simulink model "Switching_05"  (R2022b)
settings: Solver=ode4  StartTime=0.0  StopTime=50  FixedStep=1e-3  MaxStep=1e-3  RelTol=1e-3
undefined symbols (not defined in the file or in its folder): OF_b, OF_k1, OF_k2, p1, p2, p3, PR_k1, PR_k2, PR_k3, theta_d, tolerance_posture, v_sat, w_sat, x_d, y_d
libraries: simulink x18, dspsigops x3
settings Model: Creator=david  LastModifiedBy=david

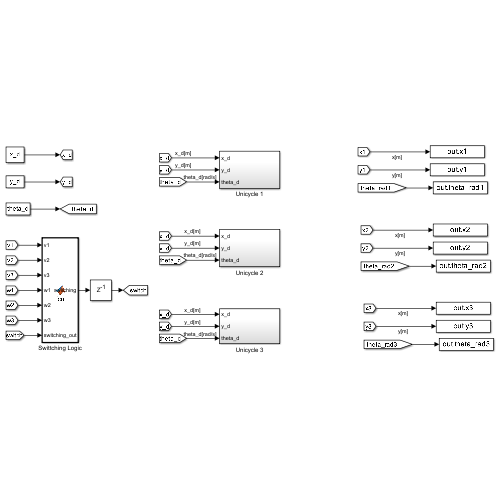
[thumbnail: Simulink's stored preview of the top-level diagram]
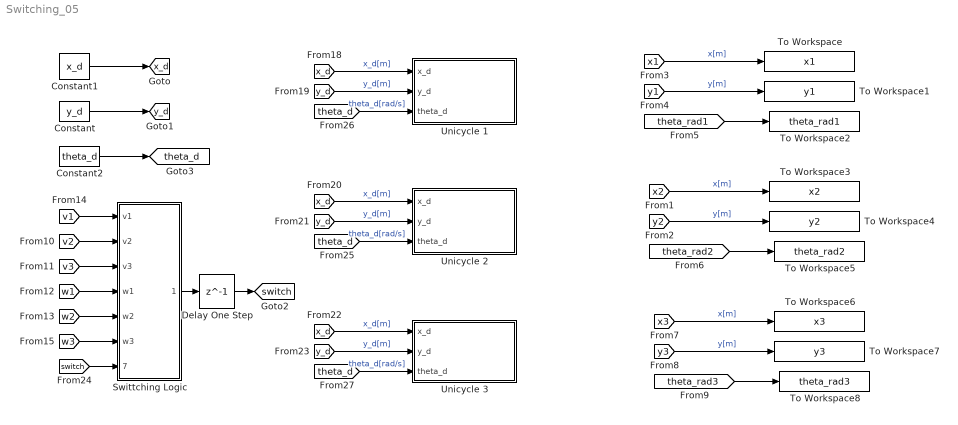
== system Switching_05 ==
  Constant : Constant  Value=y_d
  Constant1 : Constant  Value=x_d
  Constant2 : Constant  Value=theta_d
  Delay One Step : Delay  DelayLength=1
  Swittching Logic : MATLAB Function  TreatAsAtomicUnit=on
  To Workspace : ToWorkspace  VariableName=x1  SaveFormat=Structure With Time  SampleTime=-1
  To Workspace1 : ToWorkspace  VariableName=y1  SaveFormat=Structure With Time  SampleTime=-1
  To Workspace2 : ToWorkspace  VariableName=theta_rad1  SaveFormat=Structure With Time  SampleTime=-1
  To Workspace3 : ToWorkspace  VariableName=x2  SaveFormat=Structure With Time  SampleTime=-1
  To Workspace4 : ToWorkspace  VariableName=y2  SaveFormat=Structure With Time  SampleTime=-1
  To Workspace5 : ToWorkspace  VariableName=theta_rad2  SaveFormat=Structure With Time  SampleTime=-1
  To Workspace6 : ToWorkspace  VariableName=x3  SaveFormat=Structure With Time  SampleTime=-1
  To Workspace7 : ToWorkspace  VariableName=y3  SaveFormat=Structure With Time  SampleTime=-1
  To Workspace8 : ToWorkspace  VariableName=theta_rad3  SaveFormat=Structure With Time  SampleTime=-1
  Unicycle 1 : Subsystem
  Unicycle 2 : Subsystem
  Unicycle 3 : Subsystem
  tag scope: switch=global, theta_d=global, x_d=global, y_d=global
  wires:
  [x1] -> To Workspace/1  "x[m]"
  [y1] -> To Workspace1/1  "y[m]"
  [theta_rad1] -> To Workspace2/1
  [x2] -> To Workspace3/1  "x[m]"
  [y2] -> To Workspace4/1  "y[m]"
  [theta_rad2] -> To Workspace5/1
  [theta_rad3] -> To Workspace8/1
  [y3] -> To Workspace7/1  "y[m]"
  [x3] -> To Workspace6/1  "x[m]"
  Constant1/1 -> [x_d]
  Constant/1 -> [y_d]
  [x_d] -> Unicycle 1/1(x_d)  "x_d[m]"
  [y_d] -> Unicycle 1/2(y_d)  "y_d[m]"
  [y_d] -> Unicycle 2/2(y_d)  "y_d[m]"
  [x_d] -> Unicycle 2/1(x_d)  "x_d[m]"
  [y_d] -> Unicycle 3/2(y_d)  "y_d[m]"
  [x_d] -> Unicycle 3/1(x_d)  "x_d[m]"
  Swittching Logic/1(switching) -> Delay One Step/1
  [switch] -> Swittching Logic/7(switching_out)
  Delay One Step/1 -> [switch]
  Constant2/1 -> [theta_d]
  [theta_d] -> Unicycle 2/3(theta_d)  "theta_d[rad/s]"
  [theta_d] -> Unicycle 1/3(theta_d)  "theta_d[rad/s]"
  [theta_d] -> Unicycle 3/3(theta_d)  "theta_d[rad/s]"
  [w3] -> Swittching Logic/6(w3)
  [v3] -> Swittching Logic/3(v3)
  [w1] -> Swittching Logic/4(w1)
  [w2] -> Swittching Logic/5(w2)
  [v2] -> Swittching Logic/2(v2)
  [v1] -> Swittching Logic/1(v1)

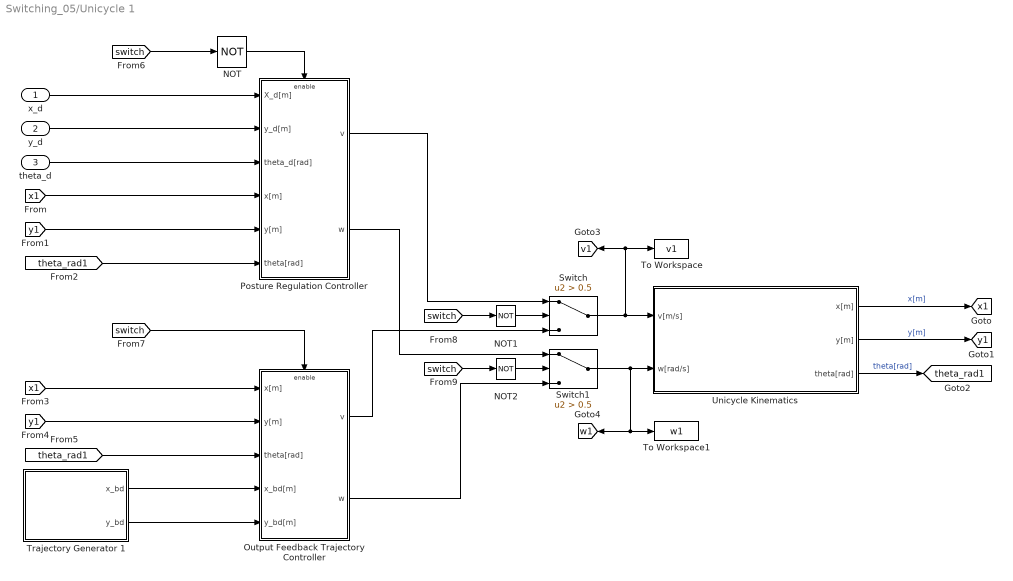
== system Switching_05/Unicycle 1 ==
  x_d : Inport
  y_d : Inport  Port=2
  theta_d : Inport  Port=3
  NOT : Logic  Operator=NOT  IconShape=distinctive  AllPortsSameDT=off  OutDataTypeStr=boolean
  NOT1 : Logic  Operator=NOT  IconShape=distinctive  AllPortsSameDT=off  OutDataTypeStr=boolean
  NOT2 : Logic  Operator=NOT  IconShape=distinctive  AllPortsSameDT=off  OutDataTypeStr=boolean
  Output Feedback Trajectory Controller : Subsystem
  Posture Regulation Controller : Subsystem
  Switch : Switch  Criteria=u2 > Threshold  Threshold=0.5  SaturateOnIntegerOverflow=off  InputSameDT=off
  Switch1 : Switch  Criteria=u2 > Threshold  Threshold=0.5  SaturateOnIntegerOverflow=off  InputSameDT=off
  To Workspace : ToWorkspace  VariableName=v1  SaveFormat=Structure With Time  SampleTime=-1
  To Workspace1 : ToWorkspace  VariableName=w1  SaveFormat=Structure With Time  SampleTime=-1
  Trajectory Generator 1 : Subsystem
  Unicycle Kinematics : Subsystem
  tag scope: theta_rad1=global, v1=global, w1=global, x1=global, y1=global
  wires:
  Unicycle Kinematics/3(theta[rad]) -> [theta_rad1]  "theta[rad]"
  [y1] -> Posture Regulation Controller/5(y[m])
  [theta_rad1] -> Posture Regulation Controller/6(theta[rad])
  Unicycle Kinematics/2(y[m]) -> [y1]  "y[m]"
  [x1] -> Posture Regulation Controller/4(x[m])
  Unicycle Kinematics/1(x[m]) -> [x1]  "x[m]"
  x_d/1 -> Posture Regulation Controller/1(X_d[m])
  y_d/1 -> Posture Regulation Controller/2(y_d[m])
  [theta_rad1] -> Output Feedback Trajectory Controller/3(theta[rad])
  [x1] -> Output Feedback Trajectory Controller/1(x[m])
  [y1] -> Output Feedback Trajectory Controller/2(y[m])
  NOT/1 -> Posture Regulation Controller/Enable
  [switch] -> NOT/1
  [switch] -> Output Feedback Trajectory Controller/Enable
  Posture Regulation Controller/2(w) -> Switch1/1
  Posture Regulation Controller/1(v) -> Switch/1
  Output Feedback Trajectory Controller/2(w) -> Switch1/3
  [switch] -> NOT2/1
  Output Feedback Trajectory Controller/1(v) -> Switch/3
  [switch] -> NOT1/1
  NOT1/1 -> Switch/2
  NOT2/1 -> Switch1/2
  Switch1/1 -> Unicycle Kinematics/2(w[rad/s]), To Workspace1/1, [w1]
  Switch/1 -> Unicycle Kinematics/1(v[m/s]), To Workspace/1, [v1]
  theta_d/1 -> Posture Regulation Controller/3(theta_d[rad])
  Trajectory Generator 1/1(x_bd) -> Output Feedback Trajectory Controller/4(x_bd[m])
  Trajectory Generator 1/2(y_bd) -> Output Feedback Trajectory Controller/5(y_bd[m])

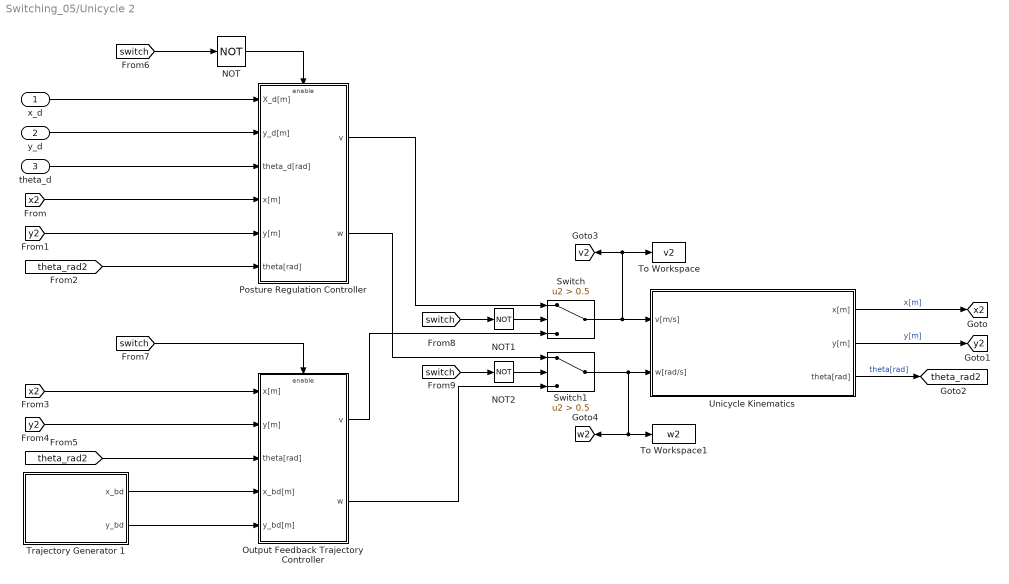
== system Switching_05/Unicycle 2 ==
  x_d : Inport
  y_d : Inport  Port=2
  theta_d : Inport  Port=3
  NOT : Logic  Operator=NOT  IconShape=distinctive  AllPortsSameDT=off  OutDataTypeStr=boolean
  NOT1 : Logic  Operator=NOT  IconShape=distinctive  AllPortsSameDT=off  OutDataTypeStr=boolean
  NOT2 : Logic  Operator=NOT  IconShape=distinctive  AllPortsSameDT=off  OutDataTypeStr=boolean
  Output Feedback Trajectory Controller : Subsystem
  Posture Regulation Controller : Subsystem
  Switch : Switch  Criteria=u2 > Threshold  Threshold=0.5  SaturateOnIntegerOverflow=off  InputSameDT=off
  Switch1 : Switch  Criteria=u2 > Threshold  Threshold=0.5  SaturateOnIntegerOverflow=off  InputSameDT=off
  To Workspace : ToWorkspace  VariableName=v2  SaveFormat=Structure With Time  SampleTime=-1
  To Workspace1 : ToWorkspace  VariableName=w2  SaveFormat=Structure With Time  SampleTime=-1
  Trajectory Generator 1 : Subsystem
  Unicycle Kinematics : Subsystem
  tag scope: theta_rad2=global, v2=global, w2=global, x2=global, y2=global
  wires:
  Unicycle Kinematics/3(theta[rad]) -> [theta_rad2]  "theta[rad]"
  [y2] -> Posture Regulation Controller/5(y[m])
  [theta_rad2] -> Posture Regulation Controller/6(theta[rad])
  Unicycle Kinematics/2(y[m]) -> [y2]  "y[m]"
  [x2] -> Posture Regulation Controller/4(x[m])
  Unicycle Kinematics/1(x[m]) -> [x2]  "x[m]"
  x_d/1 -> Posture Regulation Controller/1(X_d[m])
  y_d/1 -> Posture Regulation Controller/2(y_d[m])
  [theta_rad2] -> Output Feedback Trajectory Controller/3(theta[rad])
  [x2] -> Output Feedback Trajectory Controller/1(x[m])
  [y2] -> Output Feedback Trajectory Controller/2(y[m])
  NOT/1 -> Posture Regulation Controller/Enable
  [switch] -> NOT/1
  [switch] -> Output Feedback Trajectory Controller/Enable
  Posture Regulation Controller/2(w) -> Switch1/1
  Posture Regulation Controller/1(v) -> Switch/1
  Output Feedback Trajectory Controller/2(w) -> Switch1/3
  [switch] -> NOT2/1
  [switch] -> NOT1/1
  NOT1/1 -> Switch/2
  NOT2/1 -> Switch1/2
  Output Feedback Trajectory Controller/1(v) -> Switch/3
  Switch/1 -> Unicycle Kinematics/1(v[m/s]), To Workspace/1, [v2]
  theta_d/1 -> Posture Regulation Controller/3(theta_d[rad])
  Switch1/1 -> Unicycle Kinematics/2(w[rad/s]), [w2], To Workspace1/1
  Trajectory Generator 1/2(y_bd) -> Output Feedback Trajectory Controller/5(y_bd[m])
  Trajectory Generator 1/1(x_bd) -> Output Feedback Trajectory Controller/4(x_bd[m])

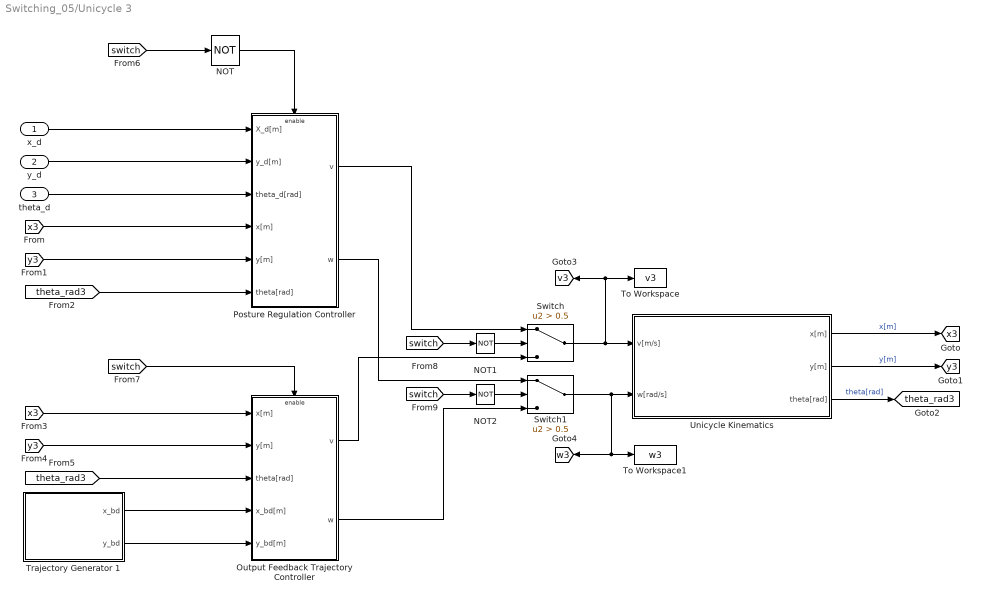
== system Switching_05/Unicycle 3 ==
  x_d : Inport
  y_d : Inport  Port=2
  theta_d : Inport  Port=3
  NOT : Logic  Operator=NOT  IconShape=distinctive  AllPortsSameDT=off  OutDataTypeStr=boolean
  NOT1 : Logic  Operator=NOT  IconShape=distinctive  AllPortsSameDT=off  OutDataTypeStr=boolean
  NOT2 : Logic  Operator=NOT  IconShape=distinctive  AllPortsSameDT=off  OutDataTypeStr=boolean
  Output Feedback Trajectory Controller : Subsystem
  Posture Regulation Controller : Subsystem
  Switch : Switch  Criteria=u2 > Threshold  Threshold=0.5  SaturateOnIntegerOverflow=off  InputSameDT=off
  Switch1 : Switch  Criteria=u2 > Threshold  Threshold=0.5  SaturateOnIntegerOverflow=off  InputSameDT=off
  To Workspace : ToWorkspace  VariableName=v3  SaveFormat=Structure With Time  SampleTime=-1
  To Workspace1 : ToWorkspace  VariableName=w3  SaveFormat=Structure With Time  SampleTime=-1
  Trajectory Generator 1 : Subsystem
  Unicycle Kinematics : Subsystem
  tag scope: theta_rad3=global, v3=global, w3=global, x3=global, y3=global
  wires:
  Unicycle Kinematics/3(theta[rad]) -> [theta_rad3]  "theta[rad]"
  [y3] -> Posture Regulation Controller/5(y[m])
  [theta_rad3] -> Posture Regulation Controller/6(theta[rad])
  Unicycle Kinematics/2(y[m]) -> [y3]  "y[m]"
  [x3] -> Posture Regulation Controller/4(x[m])
  Unicycle Kinematics/1(x[m]) -> [x3]  "x[m]"
  x_d/1 -> Posture Regulation Controller/1(X_d[m])
  y_d/1 -> Posture Regulation Controller/2(y_d[m])
  [theta_rad3] -> Output Feedback Trajectory Controller/3(theta[rad])
  [x3] -> Output Feedback Trajectory Controller/1(x[m])
  [y3] -> Output Feedback Trajectory Controller/2(y[m])
  NOT/1 -> Posture Regulation Controller/Enable
  [switch] -> NOT/1
  [switch] -> Output Feedback Trajectory Controller/Enable
  Posture Regulation Controller/1(v) -> Switch/1
  [switch] -> NOT1/1
  Output Feedback Trajectory Controller/1(v) -> Switch/3
  [switch] -> NOT2/1
  Posture Regulation Controller/2(w) -> Switch1/1
  Output Feedback Trajectory Controller/2(w) -> Switch1/3
  NOT1/1 -> Switch/2
  NOT2/1 -> Switch1/2
  Switch1/1 -> Unicycle Kinematics/2(w[rad/s]), To Workspace1/1, [w3]
  Switch/1 -> Unicycle Kinematics/1(v[m/s]), To Workspace/1, [v3]
  theta_d/1 -> Posture Regulation Controller/3(theta_d[rad])
  Trajectory Generator 1/1(x_bd) -> Output Feedback Trajectory Controller/4(x_bd[m])
  Trajectory Generator 1/2(y_bd) -> Output Feedback Trajectory Controller/5(y_bd[m])

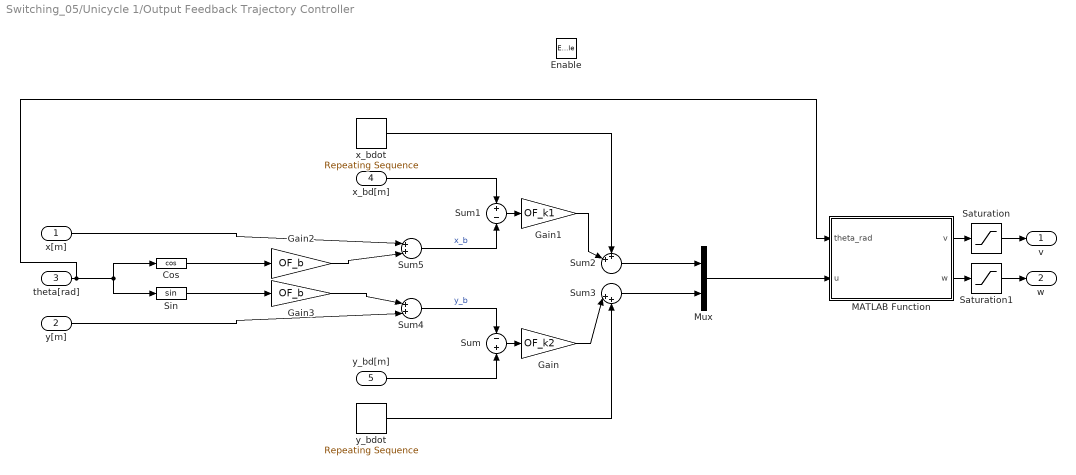
== system Switching_05/Unicycle 1/Output Feedback Trajectory Controller ==
  x[m] : Inport
  y[m] : Inport  Port=2
  theta[rad] : Inport  Port=3
  x_bd[m] : Inport  Port=4
  y_bd[m] : Inport  Port=5
  Enable : EnablePort
  Cos : Trigonometry  Operator=cos
  Gain : Gain  Gain=OF_k2
  Gain1 : Gain  Gain=OF_k1
  Gain2 : Gain  Gain=OF_b
  Gain3 : Gain  Gain=OF_b
  MATLAB Function : MATLAB Function  TreatAsAtomicUnit=on
  Mux : Mux  Inputs=2
  Saturation : Saturate  UpperLimit=v_sat  LowerLimit=-v_sat
  Saturation1 : Saturate  UpperLimit=w_sat  LowerLimit=-w_sat
  Sin : Trigonometry
  Sum : Sum  Inputs=-+
  Sum1 : Sum  Inputs=+-
  Sum2 : Sum  Inputs=++||
  Sum3 : Sum  Inputs=||++
  Sum4 : Sum  Inputs=|++|
  Sum5 : Sum  Inputs=|++|
  x_bdot : simulink/Sources/Repeating Sequence  rep_seq_t=time  rep_seq_y=x_bdot1
  y_bdot : simulink/Sources/Repeating Sequence  rep_seq_t=time  rep_seq_y=y_bdot1
  v : Outport
  w : Outport  Port=2
  wires:
  MATLAB Function/1(v) -> Saturation/1
  MATLAB Function/2(w) -> Saturation1/1
  x_bd[m]/1 -> Sum1/1
  y_bd[m]/1 -> Sum/2
  Mux/1 -> MATLAB Function/2(u)
  Sum2/1 -> Mux/1
  Sum3/1 -> Mux/2
  Sum/1 -> Gain/1
  Sum1/1 -> Gain1/1
  y_bdot/1 -> Sum3/2
  Gain/1 -> Sum3/1
  Gain1/1 -> Sum2/2
  x_bdot/1 -> Sum2/1
  Sum4/1 -> Sum/1  "y_b"
  Sum5/1 -> Sum1/2  "x_b"
  x[m]/1 -> Sum5/1
  y[m]/1 -> Sum4/2
  Cos/1 -> Gain2/1
  Gain3/1 -> Sum4/1
  Gain2/1 -> Sum5/2
  theta[rad]/1 -> Sin/1, Cos/1, MATLAB Function/1(theta_rad)
  Sin/1 -> Gain3/1
  Saturation/1 -> v/1
  Saturation1/1 -> w/1

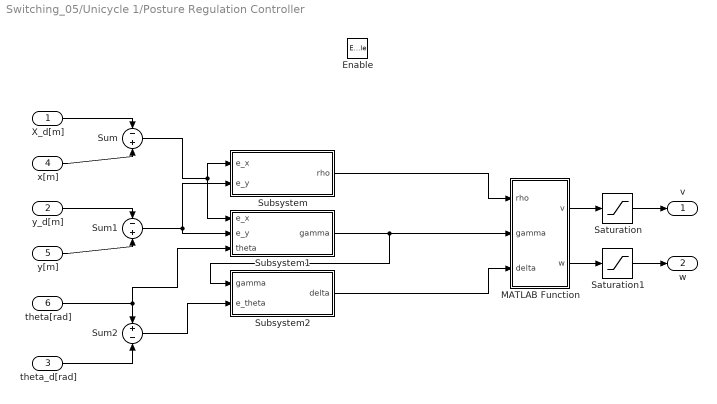
== system Switching_05/Unicycle 1/Posture Regulation Controller ==
  X_d[m] : Inport
  y_d[m] : Inport  Port=2
  theta_d[rad] : Inport  Port=3
  x[m] : Inport  Port=4
  y[m] : Inport  Port=5
  theta[rad] : Inport  Port=6
  Enable : EnablePort
  MATLAB Function : MATLAB Function  TreatAsAtomicUnit=on
  Saturation : Saturate  UpperLimit=v_sat  LowerLimit=-v_sat
  Saturation1 : Saturate  UpperLimit=w_sat  LowerLimit=-w_sat
  Subsystem : Subsystem
  Subsystem1 : Subsystem
  Subsystem2 : Subsystem
  Sum : Sum  Inputs=-+
  Sum1 : Sum  Inputs=-+
  Sum2 : Sum  Inputs=+-
  v : Outport
  w : Outport  Port=2
  wires:
  X_d[m]/1 -> Sum/1
  x[m]/1 -> Sum/2
  y_d[m]/1 -> Sum1/1
  y[m]/1 -> Sum1/2
  Sum1/1 -> Subsystem1/2(e_y), Subsystem/2(e_y)
  Sum2/1 -> Subsystem2/2(e_theta)
  Subsystem1/1(gamma) -> MATLAB Function/2(gamma), Subsystem2/1(gamma)
  Subsystem2/1(delta) -> MATLAB Function/3(delta)
  Subsystem/1(rho) -> MATLAB Function/1(rho)
  Sum/1 -> Subsystem1/1(e_x), Subsystem/1(e_x)
  MATLAB Function/1(v) -> Saturation/1
  MATLAB Function/2(w) -> Saturation1/1
  theta[rad]/1 -> Sum2/1, Subsystem1/3(theta)
  theta_d[rad]/1 -> Sum2/2
  Saturation/1 -> v/1
  Saturation1/1 -> w/1

== system Switching_05/Unicycle 1/Trajectory Generator 1 ==
  To Workspace : ToWorkspace  VariableName=x_bd1  SaveFormat=Structure With Time  SampleTime=-1
  To Workspace1 : ToWorkspace  VariableName=y_bd1  SaveFormat=Structure With Time  SampleTime=-1
  To Workspace2 : ToWorkspace  VariableName=y_d1  SaveFormat=Structure With Time  SampleTime=-1
  To Workspace3 : ToWorkspace  VariableName=x_d1  SaveFormat=Structure With Time  SampleTime=-1
  x_bd1 : simulink/Sources/Repeating Sequence  rep_seq_t=time  rep_seq_y=x_bd1
  x_d1 : simulink/Sources/Repeating Sequence  rep_seq_t=time  rep_seq_y=x_d1
  y_bd1 : simulink/Sources/Repeating Sequence  rep_seq_t=time  rep_seq_y=y_bd1
  y_d1 : simulink/Sources/Repeating Sequence  rep_seq_t=time  rep_seq_y=y_d1
  x_bd : Outport
  y_bd : Outport  Port=2
  wires:
  x_bd1/1 -> x_bd/1, To Workspace/1
  x_d1/1 -> To Workspace3/1
  y_bd1/1 -> y_bd/1, To Workspace1/1
  y_d1/1 -> To Workspace2/1

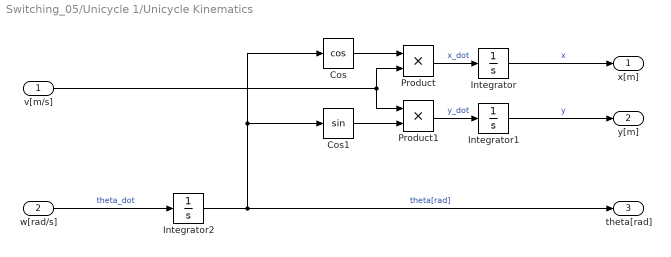
== system Switching_05/Unicycle 1/Unicycle Kinematics ==
  v[m/s] : Inport
  w[rad/s] : Inport  Port=2
  Cos : Trigonometry  Operator=cos
  Cos1 : Trigonometry
  Integrator : Integrator  InitialCondition=p1(1)
  Integrator1 : Integrator  InitialCondition=p1(2)
  Integrator2 : Integrator  InitialCondition=p1(3)
  Product : Product
  Product1 : Product
  x[m] : Outport
  y[m] : Outport  Port=2
  theta[rad] : Outport  Port=3
  wires:
  Integrator/1 -> x[m]/1  "x"
  Integrator1/1 -> y[m]/1  "y"
  w[rad/s]/1 -> Integrator2/1  "theta_dot"
  Integrator2/1 -> Cos/1, Cos1/1, theta[rad]/1  "theta[rad]"
  Product/1 -> Integrator/1  "x_dot"
  Cos1/1 -> Product1/2
  Cos/1 -> Product/1
  v[m/s]/1 -> Product1/1, Product/2
  Product1/1 -> Integrator1/1  "y_dot"

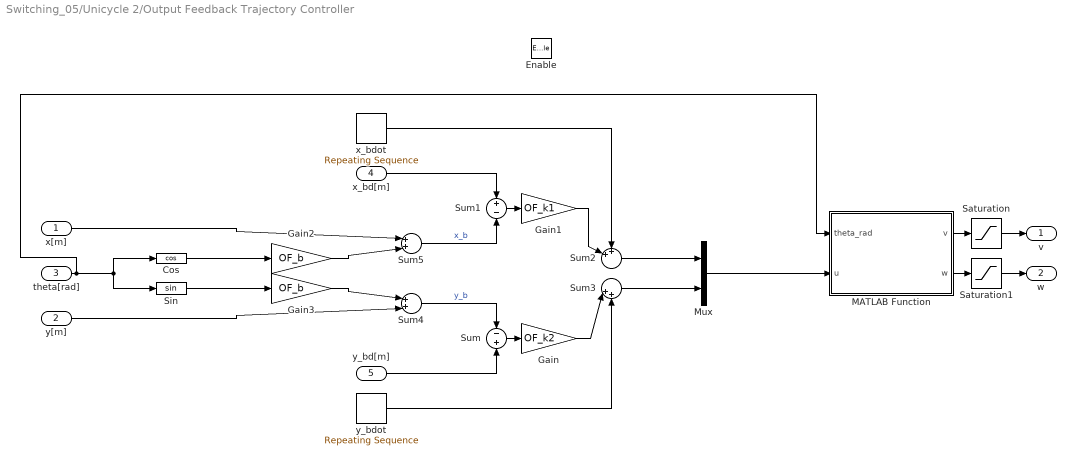
== system Switching_05/Unicycle 2/Output Feedback Trajectory Controller ==
  x[m] : Inport
  y[m] : Inport  Port=2
  theta[rad] : Inport  Port=3
  x_bd[m] : Inport  Port=4
  y_bd[m] : Inport  Port=5
  Enable : EnablePort
  Cos : Trigonometry  Operator=cos
  Gain : Gain  Gain=OF_k2
  Gain1 : Gain  Gain=OF_k1
  Gain2 : Gain  Gain=OF_b
  Gain3 : Gain  Gain=OF_b
  MATLAB Function : MATLAB Function  TreatAsAtomicUnit=on
  Mux : Mux  Inputs=2
  Saturation : Saturate  UpperLimit=v_sat  LowerLimit=-v_sat
  Saturation1 : Saturate  UpperLimit=w_sat  LowerLimit=-w_sat
  Sin : Trigonometry
  Sum : Sum  Inputs=-+
  Sum1 : Sum  Inputs=+-
  Sum2 : Sum  Inputs=++||
  Sum3 : Sum  Inputs=||++
  Sum4 : Sum  Inputs=|++|
  Sum5 : Sum  Inputs=|++|
  x_bdot : simulink/Sources/Repeating Sequence  rep_seq_t=time  rep_seq_y=x_bdot2
  y_bdot : simulink/Sources/Repeating Sequence  rep_seq_t=time  rep_seq_y=y_bdot2
  v : Outport
  w : Outport  Port=2
  wires:
  MATLAB Function/1(v) -> Saturation/1
  MATLAB Function/2(w) -> Saturation1/1
  x_bd[m]/1 -> Sum1/1
  y_bd[m]/1 -> Sum/2
  Mux/1 -> MATLAB Function/2(u)
  Sum2/1 -> Mux/1
  Sum3/1 -> Mux/2
  Sum/1 -> Gain/1
  Sum1/1 -> Gain1/1
  y_bdot/1 -> Sum3/2
  Gain/1 -> Sum3/1
  Gain1/1 -> Sum2/2
  x_bdot/1 -> Sum2/1
  Sum4/1 -> Sum/1  "y_b"
  Sum5/1 -> Sum1/2  "x_b"
  x[m]/1 -> Sum5/1
  y[m]/1 -> Sum4/2
  Cos/1 -> Gain2/1
  Gain3/1 -> Sum4/1
  Gain2/1 -> Sum5/2
  theta[rad]/1 -> Sin/1, Cos/1, MATLAB Function/1(theta_rad)
  Sin/1 -> Gain3/1
  Saturation1/1 -> w/1
  Saturation/1 -> v/1

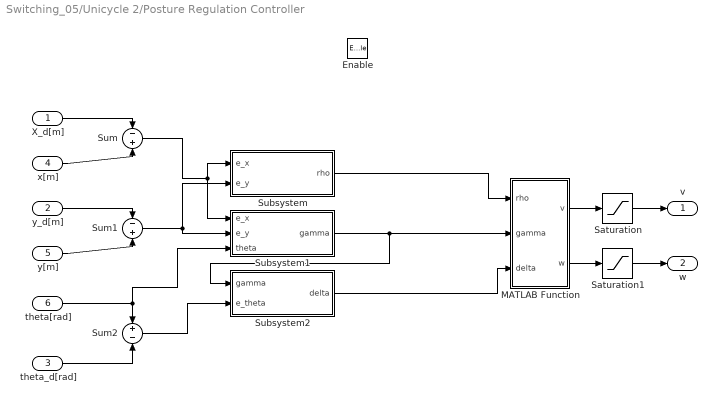
== system Switching_05/Unicycle 2/Posture Regulation Controller ==
  X_d[m] : Inport
  y_d[m] : Inport  Port=2
  theta_d[rad] : Inport  Port=3
  x[m] : Inport  Port=4
  y[m] : Inport  Port=5
  theta[rad] : Inport  Port=6
  Enable : EnablePort
  MATLAB Function : MATLAB Function  TreatAsAtomicUnit=on
  Saturation : Saturate  UpperLimit=v_sat  LowerLimit=-v_sat
  Saturation1 : Saturate  UpperLimit=w_sat  LowerLimit=-w_sat
  Subsystem : Subsystem
  Subsystem1 : Subsystem
  Subsystem2 : Subsystem
  Sum : Sum  Inputs=-+
  Sum1 : Sum  Inputs=-+
  Sum2 : Sum  Inputs=+-
  v : Outport
  w : Outport  Port=2
  wires:
  X_d[m]/1 -> Sum/1
  x[m]/1 -> Sum/2
  y_d[m]/1 -> Sum1/1
  y[m]/1 -> Sum1/2
  Sum1/1 -> Subsystem1/2(e_y), Subsystem/2(e_y)
  Sum2/1 -> Subsystem2/2(e_theta)
  Subsystem1/1(gamma) -> MATLAB Function/2(gamma), Subsystem2/1(gamma)
  Subsystem2/1(delta) -> MATLAB Function/3(delta)
  Subsystem/1(rho) -> MATLAB Function/1(rho)
  Sum/1 -> Subsystem1/1(e_x), Subsystem/1(e_x)
  MATLAB Function/1(v) -> Saturation/1
  MATLAB Function/2(w) -> Saturation1/1
  theta[rad]/1 -> Sum2/1, Subsystem1/3(theta)
  theta_d[rad]/1 -> Sum2/2
  Saturation/1 -> v/1
  Saturation1/1 -> w/1

== system Switching_05/Unicycle 2/Trajectory Generator 1 ==
  To Workspace : ToWorkspace  VariableName=x_bd2  SaveFormat=Structure With Time  SampleTime=-1
  To Workspace1 : ToWorkspace  VariableName=y_bd2  SaveFormat=Structure With Time  SampleTime=-1
  To Workspace2 : ToWorkspace  VariableName=y_d2  SaveFormat=Structure With Time  SampleTime=-1
  To Workspace3 : ToWorkspace  VariableName=x_d2  SaveFormat=Structure With Time  SampleTime=-1
  x_bd2 : simulink/Sources/Repeating Sequence  rep_seq_t=time  rep_seq_y=x_bd2
  x_d2 : simulink/Sources/Repeating Sequence  rep_seq_t=time  rep_seq_y=x_d2
  y_bd2 : simulink/Sources/Repeating Sequence  rep_seq_t=time  rep_seq_y=y_bd2
  y_d2 : simulink/Sources/Repeating Sequence  rep_seq_t=time  rep_seq_y=y_d2
  x_bd : Outport
  y_bd : Outport  Port=2
  wires:
  x_bd2/1 -> x_bd/1, To Workspace/1
  x_d2/1 -> To Workspace3/1
  y_bd2/1 -> y_bd/1, To Workspace1/1
  y_d2/1 -> To Workspace2/1

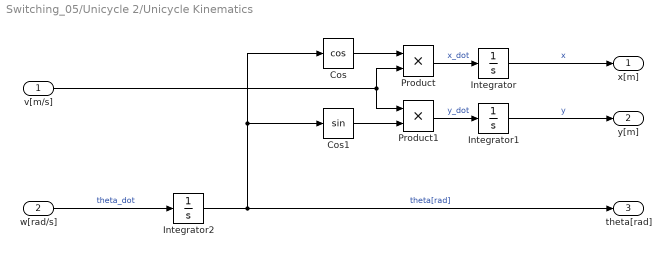
== system Switching_05/Unicycle 2/Unicycle Kinematics ==
  v[m/s] : Inport
  w[rad/s] : Inport  Port=2
  Cos : Trigonometry  Operator=cos
  Cos1 : Trigonometry
  Integrator : Integrator  InitialCondition=p2(1)
  Integrator1 : Integrator  InitialCondition=p2(2)
  Integrator2 : Integrator  InitialCondition=p2(3)
  Product : Product
  Product1 : Product
  x[m] : Outport
  y[m] : Outport  Port=2
  theta[rad] : Outport  Port=3
  wires:
  Integrator/1 -> x[m]/1  "x"
  Integrator1/1 -> y[m]/1  "y"
  w[rad/s]/1 -> Integrator2/1  "theta_dot"
  Integrator2/1 -> Cos/1, Cos1/1, theta[rad]/1  "theta[rad]"
  Product/1 -> Integrator/1  "x_dot"
  Cos1/1 -> Product1/2
  Cos/1 -> Product/1
  v[m/s]/1 -> Product1/1, Product/2
  Product1/1 -> Integrator1/1  "y_dot"

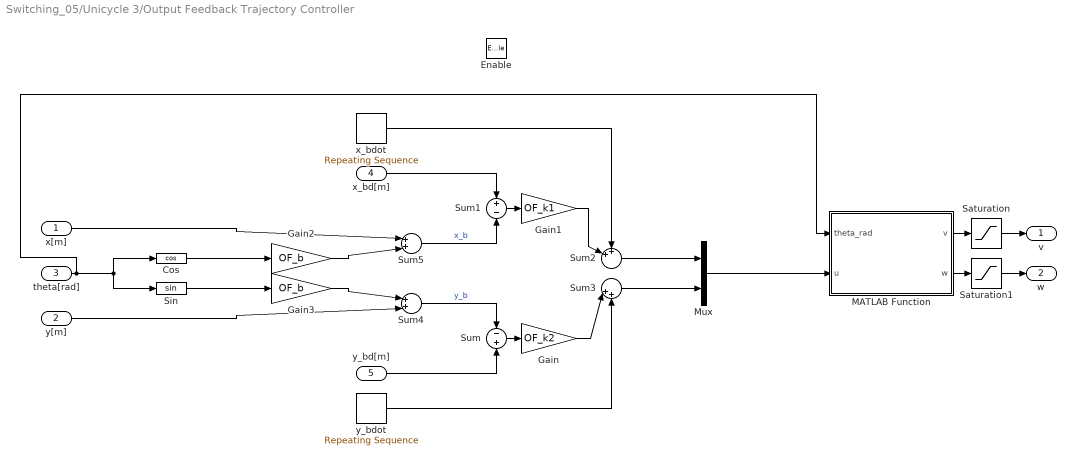
== system Switching_05/Unicycle 3/Output Feedback Trajectory Controller ==
  x[m] : Inport
  y[m] : Inport  Port=2
  theta[rad] : Inport  Port=3
  x_bd[m] : Inport  Port=4
  y_bd[m] : Inport  Port=5
  Enable : EnablePort
  Cos : Trigonometry  Operator=cos
  Gain : Gain  Gain=OF_k2
  Gain1 : Gain  Gain=OF_k1
  Gain2 : Gain  Gain=OF_b
  Gain3 : Gain  Gain=OF_b
  MATLAB Function : MATLAB Function  TreatAsAtomicUnit=on
  Mux : Mux  Inputs=2
  Saturation : Saturate  UpperLimit=v_sat  LowerLimit=-v_sat
  Saturation1 : Saturate  UpperLimit=w_sat  LowerLimit=-w_sat
  Sin : Trigonometry
  Sum : Sum  Inputs=-+
  Sum1 : Sum  Inputs=+-
  Sum2 : Sum  Inputs=++||
  Sum3 : Sum  Inputs=||++
  Sum4 : Sum  Inputs=|++|
  Sum5 : Sum  Inputs=|++|
  x_bdot : simulink/Sources/Repeating Sequence  rep_seq_t=time  rep_seq_y=x_bdot3
  y_bdot : simulink/Sources/Repeating Sequence  rep_seq_t=time  rep_seq_y=y_bdot3
  v : Outport
  w : Outport  Port=2
  wires:
  MATLAB Function/1(v) -> Saturation/1
  MATLAB Function/2(w) -> Saturation1/1
  x_bd[m]/1 -> Sum1/1
  y_bd[m]/1 -> Sum/2
  Mux/1 -> MATLAB Function/2(u)
  Sum2/1 -> Mux/1
  Sum3/1 -> Mux/2
  Sum/1 -> Gain/1
  Sum1/1 -> Gain1/1
  y_bdot/1 -> Sum3/2
  Gain/1 -> Sum3/1
  Gain1/1 -> Sum2/2
  x_bdot/1 -> Sum2/1
  Sum4/1 -> Sum/1  "y_b"
  Sum5/1 -> Sum1/2  "x_b"
  x[m]/1 -> Sum5/1
  y[m]/1 -> Sum4/2
  Cos/1 -> Gain2/1
  Gain3/1 -> Sum4/1
  Gain2/1 -> Sum5/2
  theta[rad]/1 -> Sin/1, Cos/1, MATLAB Function/1(theta_rad)
  Sin/1 -> Gain3/1
  Saturation/1 -> v/1
  Saturation1/1 -> w/1

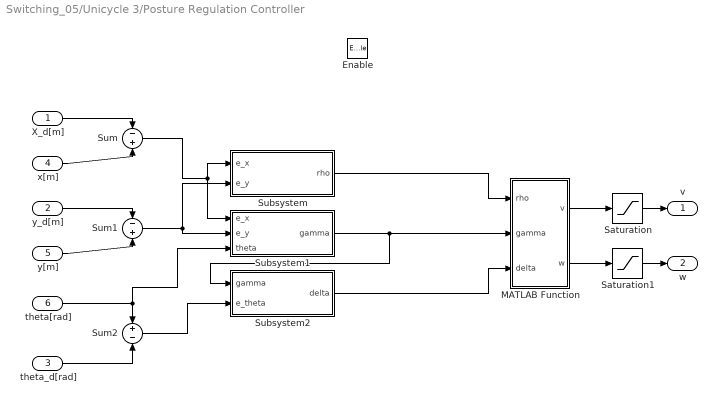
== system Switching_05/Unicycle 3/Posture Regulation Controller ==
  X_d[m] : Inport
  y_d[m] : Inport  Port=2
  theta_d[rad] : Inport  Port=3
  x[m] : Inport  Port=4
  y[m] : Inport  Port=5
  theta[rad] : Inport  Port=6
  Enable : EnablePort
  MATLAB Function : MATLAB Function  TreatAsAtomicUnit=on
  Saturation : Saturate  UpperLimit=v_sat  LowerLimit=-v_sat
  Saturation1 : Saturate  UpperLimit=w_sat  LowerLimit=-w_sat
  Subsystem : Subsystem
  Subsystem1 : Subsystem
  Subsystem2 : Subsystem
  Sum : Sum  Inputs=-+
  Sum1 : Sum  Inputs=-+
  Sum2 : Sum  Inputs=+-
  v : Outport
  w : Outport  Port=2
  wires:
  X_d[m]/1 -> Sum/1
  x[m]/1 -> Sum/2
  y_d[m]/1 -> Sum1/1
  y[m]/1 -> Sum1/2
  Sum1/1 -> Subsystem1/2(e_y), Subsystem/2(e_y)
  Sum2/1 -> Subsystem2/2(e_theta)
  Subsystem1/1(gamma) -> MATLAB Function/2(gamma), Subsystem2/1(gamma)
  Subsystem2/1(delta) -> MATLAB Function/3(delta)
  Subsystem/1(rho) -> MATLAB Function/1(rho)
  Sum/1 -> Subsystem1/1(e_x), Subsystem/1(e_x)
  MATLAB Function/1(v) -> Saturation/1
  MATLAB Function/2(w) -> Saturation1/1
  theta[rad]/1 -> Sum2/1, Subsystem1/3(theta)
  theta_d[rad]/1 -> Sum2/2
  Saturation/1 -> v/1
  Saturation1/1 -> w/1

== system Switching_05/Unicycle 3/Trajectory Generator 1 ==
  To Workspace : ToWorkspace  VariableName=x_bd3  SaveFormat=Structure With Time  SampleTime=-1
  To Workspace1 : ToWorkspace  VariableName=y_bd3  SaveFormat=Structure With Time  SampleTime=-1
  To Workspace2 : ToWorkspace  VariableName=y_d3  SaveFormat=Structure With Time  SampleTime=-1
  To Workspace3 : ToWorkspace  VariableName=x_d3  SaveFormat=Structure With Time  SampleTime=-1
  x_bd3 : simulink/Sources/Repeating Sequence  rep_seq_t=time  rep_seq_y=x_bd3
  x_d3 : simulink/Sources/Repeating Sequence  rep_seq_t=time  rep_seq_y=x_d3
  y_bd3 : simulink/Sources/Repeating Sequence  rep_seq_t=time  rep_seq_y=y_bd3
  y_d3 : simulink/Sources/Repeating Sequence  rep_seq_t=time  rep_seq_y=y_d3
  x_bd : Outport
  y_bd : Outport  Port=2
  wires:
  x_bd3/1 -> x_bd/1, To Workspace/1
  x_d3/1 -> To Workspace3/1
  y_bd3/1 -> y_bd/1, To Workspace1/1
  y_d3/1 -> To Workspace2/1

== system Switching_05/Unicycle 3/Unicycle Kinematics ==
  v[m/s] : Inport
  w[rad/s] : Inport  Port=2
  Cos : Trigonometry  Operator=cos
  Cos1 : Trigonometry
  Integrator : Integrator  InitialCondition=p3(1)
  Integrator1 : Integrator  InitialCondition=p3(2)
  Integrator2 : Integrator  InitialCondition=p3(3)
  Product : Product
  Product1 : Product
  x[m] : Outport
  y[m] : Outport  Port=2
  theta[rad] : Outport  Port=3
  wires:
  Integrator/1 -> x[m]/1  "x"
  Integrator1/1 -> y[m]/1  "y"
  w[rad/s]/1 -> Integrator2/1  "theta_dot"
  Integrator2/1 -> Cos/1, Cos1/1, theta[rad]/1  "theta[rad]"
  Product/1 -> Integrator/1  "x_dot"
  Cos1/1 -> Product1/2
  Cos/1 -> Product/1
  v[m/s]/1 -> Product1/1, Product/2
  Product1/1 -> Integrator1/1  "y_dot"

== system Switching_05/Unicycle 1/Posture Regulation Controller/Subsystem ==
  e_x : Inport
  e_y : Inport  Port=2
  Sqrt : Sqrt
  Square : Math  Operator=square
  Square1 : Math  Operator=square
  Sum : Sum
  rho : Outport
  wires:
  Sqrt/1 -> rho/1
  e_x/1 -> Square/1
  e_y/1 -> Square1/1
  Sum/1 -> Sqrt/1
  Square/1 -> Sum/1
  Square1/1 -> Sum/2

== system Switching_05/Unicycle 1/Posture Regulation Controller/Subsystem1 ==
  e_x : Inport
  e_y : Inport  Port=2
  theta : Inport  Port=3
  Atan2 : Trigonometry  Operator=atan2
  Constant : Constant  Value=pi
  Sum : Sum  Inputs=+-+
  Unwrap : dspsigops/Unwrap  tol=pi  InputProcessing=Columns as channels (frame based)  running=off
  gamma : Outport
  wires:
  e_x/1 -> Atan2/2
  e_y/1 -> Atan2/1
  theta/1 -> Sum/2
  Sum/1 -> gamma/1
  Atan2/1 -> Unwrap/1
  Constant/1 -> Sum/3
  Unwrap/1 -> Sum/1

== system Switching_05/Unicycle 1/Posture Regulation Controller/Subsystem2 ==
  gamma : Inport
  e_theta : Inport  Port=2
  Sum : Sum
  delta : Outport
  wires:
  e_theta/1 -> Sum/2
  Sum/1 -> delta/1
  gamma/1 -> Sum/1

== system Switching_05/Unicycle 2/Posture Regulation Controller/Subsystem ==
  e_x : Inport
  e_y : Inport  Port=2
  Sqrt : Sqrt
  Square : Math  Operator=square
  Square1 : Math  Operator=square
  Sum : Sum
  rho : Outport
  wires:
  Sqrt/1 -> rho/1
  e_x/1 -> Square/1
  e_y/1 -> Square1/1
  Sum/1 -> Sqrt/1
  Square/1 -> Sum/1
  Square1/1 -> Sum/2

== system Switching_05/Unicycle 2/Posture Regulation Controller/Subsystem1 ==
  e_x : Inport
  e_y : Inport  Port=2
  theta : Inport  Port=3
  Atan2 : Trigonometry  Operator=atan2
  Constant : Constant  Value=pi
  Sum : Sum  Inputs=+-+
  Unwrap : dspsigops/Unwrap  tol=pi  InputProcessing=Columns as channels (frame based)  running=off
  gamma : Outport
  wires:
  e_x/1 -> Atan2/2
  e_y/1 -> Atan2/1
  theta/1 -> Sum/2
  Sum/1 -> gamma/1
  Atan2/1 -> Unwrap/1
  Constant/1 -> Sum/3
  Unwrap/1 -> Sum/1

== system Switching_05/Unicycle 2/Posture Regulation Controller/Subsystem2 ==
  gamma : Inport
  e_theta : Inport  Port=2
  Sum : Sum
  delta : Outport
  wires:
  e_theta/1 -> Sum/2
  Sum/1 -> delta/1
  gamma/1 -> Sum/1

== system Switching_05/Unicycle 3/Posture Regulation Controller/Subsystem ==
  e_x : Inport
  e_y : Inport  Port=2
  Sqrt : Sqrt
  Square : Math  Operator=square
  Square1 : Math  Operator=square
  Sum : Sum
  rho : Outport
  wires:
  Sqrt/1 -> rho/1
  e_x/1 -> Square/1
  e_y/1 -> Square1/1
  Sum/1 -> Sqrt/1
  Square/1 -> Sum/1
  Square1/1 -> Sum/2

== system Switching_05/Unicycle 3/Posture Regulation Controller/Subsystem1 ==
  e_x : Inport
  e_y : Inport  Port=2
  theta : Inport  Port=3
  Atan2 : Trigonometry  Operator=atan2
  Constant : Constant  Value=pi
  Sum : Sum  Inputs=+-+
  Unwrap : dspsigops/Unwrap  tol=pi  InputProcessing=Columns as channels (frame based)  running=off
  gamma : Outport
  wires:
  e_x/1 -> Atan2/2
  e_y/1 -> Atan2/1
  theta/1 -> Sum/2
  Sum/1 -> gamma/1
  Atan2/1 -> Unwrap/1
  Constant/1 -> Sum/3
  Unwrap/1 -> Sum/1

== system Switching_05/Unicycle 3/Posture Regulation Controller/Subsystem2 ==
  gamma : Inport
  e_theta : Inport  Port=2
  Sum : Sum
  delta : Outport
  wires:
  e_theta/1 -> Sum/2
  Sum/1 -> delta/1
  gamma/1 -> Sum/1

== matlab function Switching_05/Unicycle 2/Output Feedback Trajectory Controller/MATLAB Function ==
  data: theta_rad input; u input; v output; w output; OF_b parameter
function [v,w] = fcn(theta_rad, u, OF_b)


T_inv=[cos(theta_rad)       sin(theta_rad);
       -sin(theta_rad)/OF_b    cos(theta_rad)/OF_b];

in=T_inv*u;

v = in(1);
w= in(2);

== matlab function Switching_05/Unicycle 1/Output Feedback Trajectory Controller/MATLAB Function ==
  data: theta_rad input; u input; v output; w output; OF_b parameter
function [v,w] = fcn(theta_rad, u, OF_b)


T_inv=[cos(theta_rad)       sin(theta_rad);
       -sin(theta_rad)/OF_b    cos(theta_rad)/OF_b];

in=T_inv*u;

v = in(1);
w= in(2);

== matlab function Switching_05/Unicycle 3/Output Feedback Trajectory Controller/MATLAB Function ==
  data: theta_rad input; u input; v output; w output; OF_b parameter
function [v,w] = fcn(theta_rad, u, OF_b)


T_inv=[cos(theta_rad)       sin(theta_rad);
       -sin(theta_rad)/OF_b    cos(theta_rad)/OF_b];

in=T_inv*u;

v = in(1);
w= in(2);

== matlab function Switching_05/Swittching Logic ==
  data: switching output; v1 input; v2 input; v3 input; w1 input; w2 input; w3 input; switching_out input
function switching = fcn(v1, v2, v3, w1, w2, w3, switching_out)
if switching_out==1
    switching=1;
else
    if v1==0 && v2==0 && v3==0 && w1==0 && w2==0 && w3==0
        switching = 1; 
    else
        switching = 0; 
    end
end

== matlab function Switching_05/Unicycle 2/Posture Regulation Controller/MATLAB Function ==
  data: rho input; v output; w output; gamma input; delta input; PR_k1 parameter; PR_k2 parameter; PR_k3 parameter; tolerance_posture parameter
function [v,w] = fcn(rho, gamma, delta, PR_k1, PR_k2, PR_k3, tolerance_posture)

if abs(rho)<tolerance_posture
    v=0;
    w=0;
else
    v=PR_k1*rho*cos(gamma);
    w=PR_k2*gamma+PR_k1*(cos(gamma)*sin(gamma))/gamma*(gamma+PR_k3*delta);
end

== matlab function Switching_05/Unicycle 3/Posture Regulation Controller/MATLAB Function ==
  data: rho input; v output; w output; gamma input; delta input; PR_k1 parameter; PR_k2 parameter; PR_k3 parameter; tolerance_posture parameter
function [v,w] = fcn(rho, gamma, delta, PR_k1, PR_k2, PR_k3, tolerance_posture)

if abs(rho)<tolerance_posture
    v=0;
    w=0;
else
    v=PR_k1*rho*cos(gamma);
    w=PR_k2*gamma+PR_k1*(cos(gamma)*sin(gamma))/gamma*(gamma+PR_k3*delta);
end

== matlab function Switching_05/Unicycle 1/Posture Regulation Controller/MATLAB Function ==
  data: rho input; v output; w output; gamma input; delta input; PR_k1 parameter; PR_k2 parameter; PR_k3 parameter; tolerance_posture parameter
function [v,w] = fcn(rho, gamma, delta, PR_k1, PR_k2, PR_k3, tolerance_posture)

if abs(rho)<tolerance_posture
    v=0;
    w=0;
else
    v=PR_k1*rho*cos(gamma);
    w=PR_k2*gamma+PR_k1*(cos(gamma)*sin(gamma))/gamma*(gamma+PR_k3*delta);
end
